simulink model "Lab_Modulation_FM"  (R2021b)
settings: Solver=VariableStepAuto  StartTime=0.0  StopTime=10.0  RelTol=1e-3
libraries: dspmathops x1, commanapbnd3 x1, dspfdesign x1
settings Model: Creator=User  LastModifiedBy=aleksejshevcenko
settings SolverCC: AlgebraicLoopSolver=TrustRegion
settings DataIOCC: ReturnWorkspaceOutputs=off
settings DebuggingCC: SFMachineParentedDataDiag=warning  ArithmeticOperatorsInVariantConditions=warning
settings SFSimCC: SimUseLocalCustomCode=off  CustomCodeUndefinedFunction=UseInterfaceOnly
settings RTWCC: RTWUseLocalCustomCode=off
settings CodeAppCC: StateflowObjectComments=on

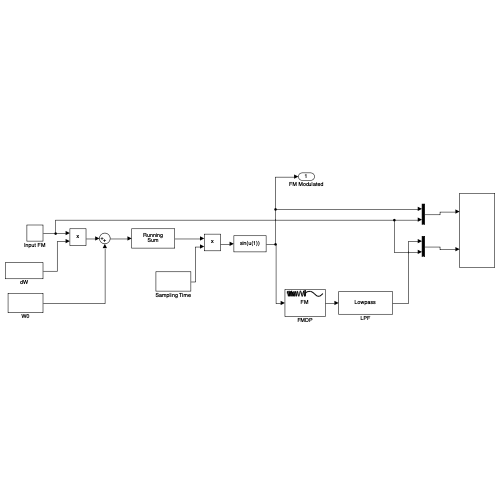
[thumbnail: Simulink's stored preview of the top-level diagram]
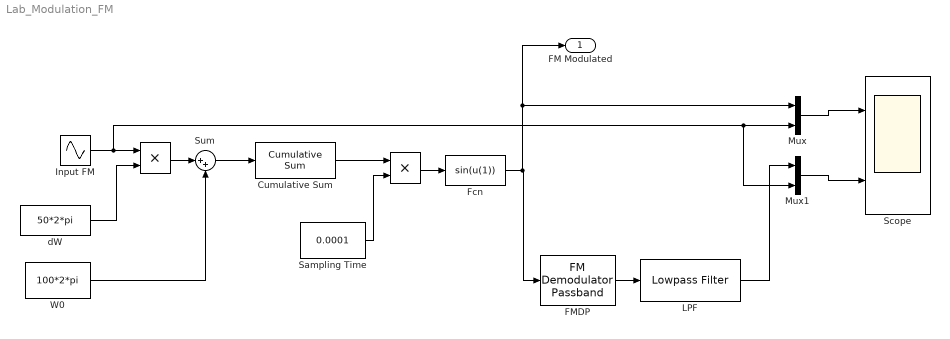
== system Lab_Modulation_FM ==
  " " : Product
  " " : Product
  Cumulative Sum : dspmathops/Cumulative Sum  dim=Channels (running sum)  reset_popup=None  roundingMode=Floor  overflowMode=off  outputDataTypeStr=Inherit: Same as accumulator  outputMin=[]  outputMax=[]  outputLastDataTypeStr=Inherit: Same as accumulator
  FMDP : commanapbnd3/FM Demodulator Passband  Fc=100  Ph=0  Kc=50  Ho=100
      settings: SourceProductBaseCode=CM
  Fcn : Fcn  Expr=sin(u(1))
  "Input FM " : Sin  Frequency=2*2*pi  SampleTime=0.0001
  "LPF " : dspfdesign/Lowpass Filter  FilterType=FIR  DesignForMinimumOrder=on  FilterOrder=50  PassbandFrequency=0.1  StopbandFrequency=100  PassbandRipple=0.1  StopbandAttenuation=80  InheritSampleRate=on  SampleRate=44100  SimulateUsing=Interpreted execution  roundingMode=Floor  coeffsDataTypeStr=fixdt(1,16)
  Mux : Mux  Inputs=2
  Mux1 : Mux  Inputs=2
  "Sampling Time " : Constant  Value=0.0001
  Scope : Scope  NumInputPorts=2
  Sum : Sum  Inputs=|++
  "W0 " : Constant  Value=100*2*pi
  dW : Constant  Value=50*2*pi
  FM Modulated : Outport
  wires:
  dW/1 -> " "/2
  "Input FM "/1 -> Mux/2, Mux1/2, " "/1
  "W0 "/1 -> Sum/2
  " "/1 -> Sum/1
  "LPF "/1 -> Mux1/1
  Mux/1 -> Scope/1
  Mux1/1 -> Scope/2
  Sum/1 -> Cumulative Sum/1
  Cumulative Sum/1 -> " "/1
  "Sampling Time "/1 -> " "/2
  " "/1 -> Fcn/1
  FMDP/1 -> "LPF "/1
  Fcn/1 -> Mux/1, FM Modulated/1, FMDP/1
